simulink model "quadcoptermodel"  (R2014b)
settings: Solver=ode45  StartTime=0.0  StopTime=10.0  RelTol=1e-3
values from neighbouring files (symbols this model uses):
  F = [zeros(2,4); c_t c_t c_t c_t]    [update_state_matrices.m]
  I = [   0.5119e-6 0 0 ... (first row only)    [update_state_matrices.m]
  M = [   d*c_t d*c_t -d*c_t -d*c_t ... (first row only)    [update_state_matrices.m]
  mass = 0.022    [update_state_matrices.m]
undefined symbols (not defined in the file or in its folder): R_30, R_31, R_32
settings Model: Creator=Mikael  LastModifiedBy=Mikael

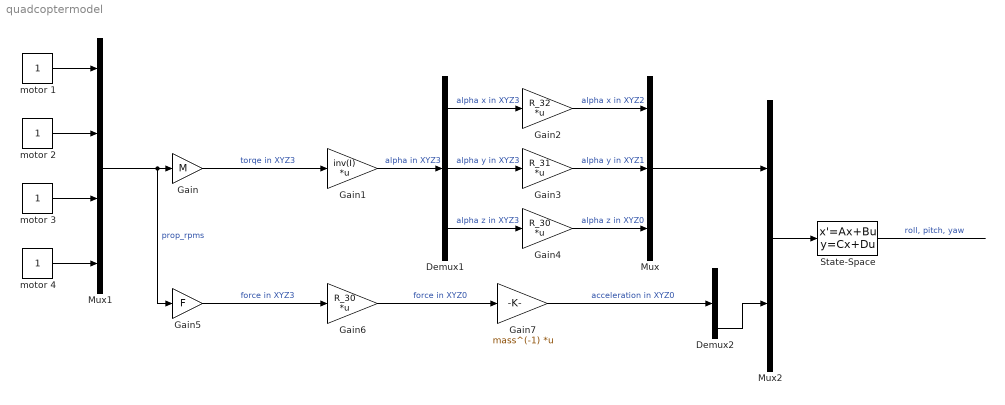
== system quadcoptermodel ==
  Demux1 : Demux  Outputs=3
  Demux2 : Demux  Outputs=3
  Gain : Gain  Gain=M
  Gain1 : Gain  Gain=inv(I)  Multiplication=Matrix(K*u) (u vector)
  Gain2 : Gain  Gain=R_32  Multiplication=Matrix(K*u) (u vector)
  Gain3 : Gain  Gain=R_31  Multiplication=Matrix(K*u) (u vector)
  Gain4 : Gain  Gain=R_30  Multiplication=Matrix(K*u) (u vector)
  Gain5 : Gain  Gain=F
  Gain6 : Gain  Gain=R_30  Multiplication=Matrix(K*u) (u vector)
  Gain7 : Gain  Gain=mass^(-1)  Multiplication=Matrix(K*u) (u vector)
  Mux : Mux  Inputs=3
  Mux1 : Mux
  Mux2 : Mux  Inputs=2
  State-Space : StateSpace  X0=0
  motor {1..4} (4 alike) : Constant
  wires:
  Gain/1 -> Gain1/1  "torqe in XYZ3"
  Gain1/1 -> Demux1/1  "alpha in XYZ3"
  Demux1/1 -> Gain2/1  "alpha x in XYZ3"
  Demux1/2 -> Gain3/1  "alpha y in XYZ3"
  Demux1/3 -> Gain4/1  "alpha z in XYZ3"
  Gain2/1 -> Mux/1  "alpha x in XYZ2"
  Gain3/1 -> Mux/2  "alpha y in XYZ1"
  Gain4/1 -> Mux/3  "alpha z in XYZ0"
  Mux/1 -> Mux2/1
  Mux1/1 -> Gain5/1, Gain/1  "prop_rpms"
  motor 1/1 -> Mux1/1
  motor 2/1 -> Mux1/2
  motor 3/1 -> Mux1/3
  motor 4/1 -> Mux1/4
  Gain5/1 -> Gain6/1  "force in XYZ3"
  Gain6/1 -> Gain7/1  "force in XYZ0"
  Gain7/1 -> Demux2/1  "acceleration in XYZ0"
  Mux2/1 -> State-Space/1
  Demux2/3 -> Mux2/2
  State-Space/1 -> ?  "roll, pitch, yaw"
